simulink model "Quadcopter_Control_Simulink"  (R2022b)
settings: Solver=VariableStepAuto  StartTime=0.0  StopTime=20  RelTol=1e-3
libraries: slpidlib x6, matrix_library x4, aerolib6dof2 x1
settings Model: Creator=matho  LastModifiedBy=matho

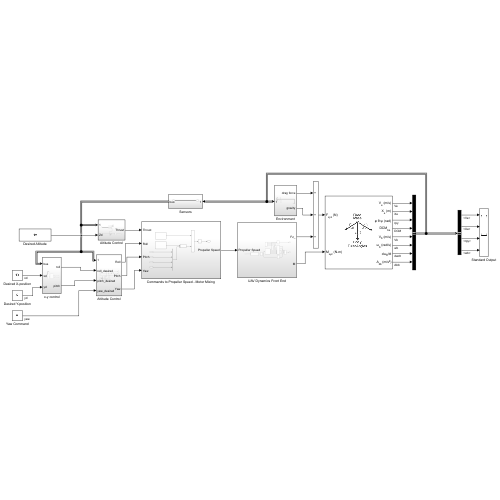
[thumbnail: Simulink's stored preview of the top-level diagram]
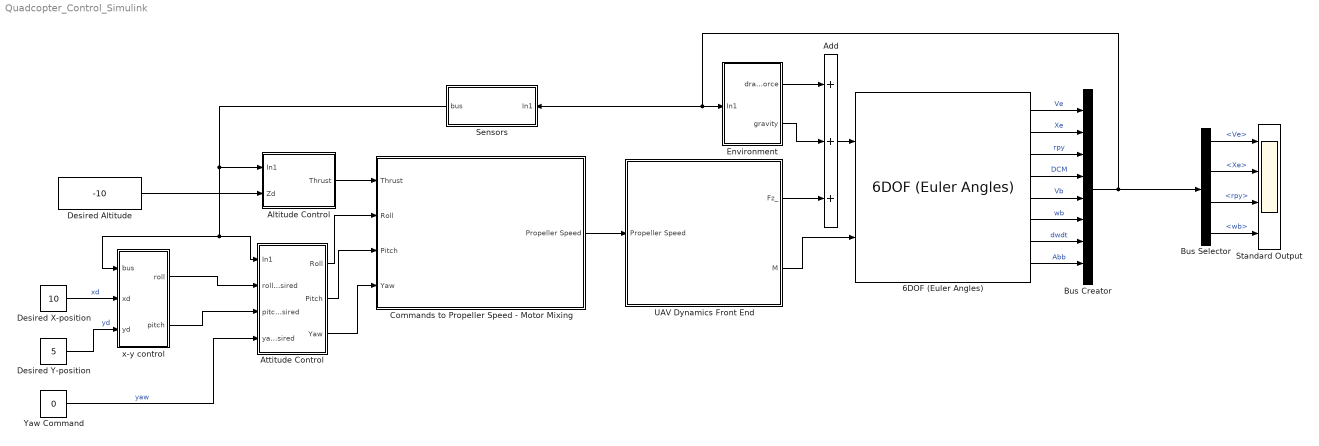
== system Quadcopter_Control_Simulink ==
  6DOF (Euler Angles) : aerolib6dof2/6DOF (Euler Angles)  units=Metric (MKS)  mtype=Fixed  rep=Euler Angles  xme_0=[0 0 0]  Vm_0=[0 0 0]  eul_0=[0 0 0]  pm_0=[0 0 0]  mass_0=1.0  mass_e=0.5  mass_f=2.0  inertia=eye(3)  inertia_e=eye(3)  inertia_f=2*eye(3)  k_quat=1.0  vre_flag=on  abi_flag=off  aMode=0  xme_statename=''  Vm_statename=''  eul_statename=''  quat_statename=''  pm_statename=''  mass_statename=''
  Add : Sum  Inputs=+++
  Altitude Control : Subsystem
  Attitude Control : Subsystem
  Bus Creator : BusCreator  Inputs=8
  Bus Selector : BusSelector  OutputSignals=Ve,Xe,rpy,wb
  "Commands to Propeller Speed - Motor Mixing " : Subsystem
  Desired Altitude : Constant  Value=-10
  Desired X-position : Constant  Value=10
  Desired Y-position : Constant  Value=5
  Environment : Subsystem
  Sensors : Subsystem
  Standard Output : Scope  NumInputPorts=4
  UAV Dynamics Front End : Subsystem
  Yaw Command : Constant  Value=0
  x-y control : Subsystem
  wires:
  6DOF (Euler Angles)/1 -> Bus Creator/1  "Ve"
  6DOF (Euler Angles)/2 -> Bus Creator/2  "Xe"
  6DOF (Euler Angles)/3 -> Bus Creator/3  "rpy"
  6DOF (Euler Angles)/4 -> Bus Creator/4  "DCM"
  6DOF (Euler Angles)/5 -> Bus Creator/5  "Vb"
  6DOF (Euler Angles)/6 -> Bus Creator/6  "wb"
  6DOF (Euler Angles)/7 -> Bus Creator/7  "dwdt"
  6DOF (Euler Angles)/8 -> Bus Creator/8  "Abb"
  Bus Selector/3 -> Standard Output/3  "<rpy>"
  Bus Selector/4 -> Standard Output/4  "<wb>"
  Bus Selector/2 -> Standard Output/2  "<Xe>"
  Bus Selector/1 -> Standard Output/1  "<Ve>"
  Add/1 -> 6DOF (Euler Angles)/1
  Bus Creator/1 -> Bus Selector/1, Sensors/1(In1), Environment/1(In1)
  Environment/1(drag force) -> Add/1
  Environment/2(gravity) -> Add/2
  UAV Dynamics Front End/2(M) -> 6DOF (Euler Angles)/2
  UAV Dynamics Front End/1(Fz_) -> Add/3
  "Commands to Propeller Speed - Motor Mixing "/1(Propeller Speed) -> UAV Dynamics Front End/1(Propeller Speed)
  Sensors/1(bus) -> Altitude Control/1(In1), Attitude Control/1(In1), x-y control/1(bus)
  Altitude Control/1(Thrust) -> "Commands to Propeller Speed - Motor Mixing "/1(Thrust)
  Attitude Control/1(Roll) -> "Commands to Propeller Speed - Motor Mixing "/2(Roll)
  Attitude Control/2(Pitch) -> "Commands to Propeller Speed - Motor Mixing "/3(Pitch)
  Attitude Control/3(Yaw) -> "Commands to Propeller Speed - Motor Mixing "/4(Yaw)
  Desired Altitude/1 -> Altitude Control/2(Zd)
  x-y control/1(roll) -> Attitude Control/2(roll_desired)
  x-y control/2(pitch) -> Attitude Control/3(pitch_desired)
  Desired X-position/1 -> x-y control/2(xd)  "xd"
  Desired Y-position/1 -> x-y control/3(yd)  "yd"
  Yaw Command/1 -> Attitude Control/4(yaw_desired)  "yaw"

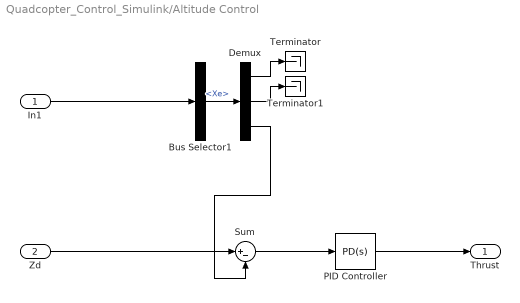
== system Quadcopter_Control_Simulink/Altitude Control ==
  In1 : Inport
  Zd : Inport  Port=2
  Bus Selector1 : BusSelector  OutputSignals=Xe
  Demux : Demux  Outputs=3
  PID Controller : slpidlib/PID Controller  Controller=PD  Form=Parallel  TimeDomain=Continuous-time  UseExternalTs=off  SampleTime=-1  IntegratorMethod=Forward Euler  FilterMethod=Forward Euler  ControllerParametersSource=internal  P=1  I=1  UseKiTs=off  D=2  N=100  UseFilter=on  TunerSelectOption=Transfer Function Based (PID Tuner App)  InitialConditionSource=internal  InitialConditionForIntegrator=0  InitialConditionForFilter=0  DifferentiatorICPrevScaledInput=0  ExternalReset=none  TrackingMode=off  Kt=1  LimitOutput=off  SatLimitsSource=internal  UpperSaturationLimit=inf  LowerSaturationLimit=-inf  LinearizeAsGain=on  AntiWindupMode=none  Kb=1  LimitIntegrator=off  UpperIntegratorSaturationLimit=inf  LowerIntegratorSaturationLimit=-inf  POutMin=[]  POutMax=[]  IOutMin=[]  IOutMax=[]  DOutMin=[]  DOutMax=[]  NOutMin=[]  NOutMax=[]  SumOutMin=[]  SumOutMax=[]  SaturationOutMin=[]  SaturationOutMax=[]  PParamMin=[]  PParamMax=[]  IParamMin=[]  IParamMax=[]  DParamMin=[]  DParamMax=[]  NParamMin=[]  NParamMax=[]  KbParamMin=[]  KbParamMax=[]  KtParamMin=[]  KtParamMax=[]  KbOutMin=[]  KbOutMax=[]  KtOutMin=[]  KtOutMax=[]  IntegratorOutMin=[]  IntegratorOutMax=[]  FilterOutMin=[]  FilterOutMax=[]  SumI1OutMin=[]  SumI1OutMax=[]  SumI2OutMin=[]  SumI2OutMax=[]  SumI3OutMin=[]  SumI3OutMax=[]  SumI4OutMin=[]  SumI4OutMax=[]  SumDOutMin=[]  SumDOutMax=[]  DifferentiatorOutMin=[]  DifferentiatorOutMax=[]  FilterDiffOutCoefMin=[]  FilterDiffOutCoefMax=[]  ReciprocalOutMin=[]  ReciprocalOutMax=[]  SumDenOutMin=[]  SumDenOutMax=[]  SumNumOutMin=[]  SumNumOutMax=[]  DivideOutMin=[]  DivideOutMax=[]  UdiffTsProdOutMin=[]  UdiffTsProdOutMax=[]  NTsProdOutMin=[]  NTsProdOutMax=[]  UintegralTsProdOutMin=[]  UintegralTsProdOutMax=[]  UngainTsProdOutMin=[]  UngainTsProdOutMax=[]  IntegratorContinuousStateAttributes=''  IntegratorStateMustResolveToSignalObject=off  IntegratorRTWStateStorageClass=Auto  FilterContinuousStateAttributes=''  FilterStateMustResolveToSignalObject=off  FilterRTWStateStorageClass=Auto  ParallelPVariant=InternalParameters  IdealPVariant=Disabled  IVariant=Disabled  DVariant=InternalParameters  IntegratorVariant=Disabled  SatVariant=Disabled  AWVariant=Disabled  PCopyVariant=Disabled  TRVariant=Disabled  FdbkBlocksVariant=Forward  IdealPFdbkVariant=Disabled  SatFdbkVariant=Disabled  DerivativeFilterVariant=ContFilter  NVariant=InternalParameters  NCopyVariant=Disabled  FilterICVariant=InternalICsFilter  IntegratorICVariant=Disabled  ExternalResetVariant=Disabled  TRSumVariant=Passthrough  SumFdbkVariant=Disabled  SumVariant=Sum_PD  TsampFilterVariant=InternalTs  TsampNgainVariant=Passthrough  TsampIntegralVariant=Disabled_SignalSpec  ExternalSaturationOutDataTypeStr=Inherit: Same as second input
  Sum : Sum  Inputs=|+-
  Terminator : Terminator
  Terminator1 : Terminator
  Thrust : Outport
  wires:
  Sum/1 -> PID Controller/1
  Demux/3 -> Sum/2
  Demux/1 -> Terminator/1
  Bus Selector1/1 -> Demux/1  "<Xe>"
  Demux/2 -> Terminator1/1
  In1/1 -> Bus Selector1/1
  PID Controller/1 -> Thrust/1
  Zd/1 -> Sum/1

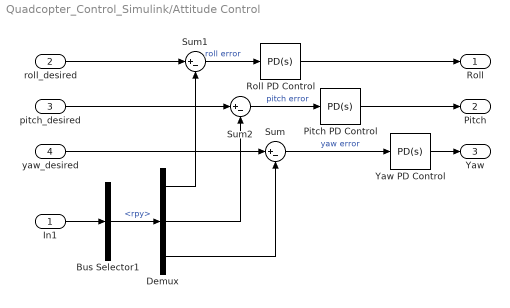
== system Quadcopter_Control_Simulink/Attitude Control ==
  In1 : Inport
  roll_desired : Inport  Port=2
  pitch_desired : Inport  Port=3
  yaw_desired : Inport  Port=4
  Bus Selector1 : BusSelector  OutputSignals=rpy
  Demux : Demux  Outputs=3
  Pitch PD Control : slpidlib/PID Controller  Controller=PD  Form=Parallel  TimeDomain=Continuous-time  UseExternalTs=off  SampleTime=-1  IntegratorMethod=Forward Euler  FilterMethod=Forward Euler  ControllerParametersSource=internal  P=1  I=1  UseKiTs=off  D=2  N=100  UseFilter=on  TunerSelectOption=Transfer Function Based (PID Tuner App)  InitialConditionSource=internal  InitialConditionForIntegrator=0  InitialConditionForFilter=0  DifferentiatorICPrevScaledInput=0  ExternalReset=none  TrackingMode=off  Kt=1  LimitOutput=off  SatLimitsSource=internal  UpperSaturationLimit=inf  LowerSaturationLimit=-inf  LinearizeAsGain=on  AntiWindupMode=none  Kb=1  LimitIntegrator=off  UpperIntegratorSaturationLimit=inf  LowerIntegratorSaturationLimit=-inf  POutMin=[]  POutMax=[]  IOutMin=[]  IOutMax=[]  DOutMin=[]  DOutMax=[]  NOutMin=[]  NOutMax=[]  SumOutMin=[]  SumOutMax=[]  SaturationOutMin=[]  SaturationOutMax=[]  PParamMin=[]  PParamMax=[]  IParamMin=[]  IParamMax=[]  DParamMin=[]  DParamMax=[]  NParamMin=[]  NParamMax=[]  KbParamMin=[]  KbParamMax=[]  KtParamMin=[]  KtParamMax=[]  KbOutMin=[]  KbOutMax=[]  KtOutMin=[]  KtOutMax=[]  IntegratorOutMin=[]  IntegratorOutMax=[]  FilterOutMin=[]  FilterOutMax=[]  SumI1OutMin=[]  SumI1OutMax=[]  SumI2OutMin=[]  SumI2OutMax=[]  SumI3OutMin=[]  SumI3OutMax=[]  SumI4OutMin=[]  SumI4OutMax=[]  SumDOutMin=[]  SumDOutMax=[]  DifferentiatorOutMin=[]  DifferentiatorOutMax=[]  FilterDiffOutCoefMin=[]  FilterDiffOutCoefMax=[]  ReciprocalOutMin=[]  ReciprocalOutMax=[]  SumDenOutMin=[]  SumDenOutMax=[]  SumNumOutMin=[]  SumNumOutMax=[]  DivideOutMin=[]  DivideOutMax=[]  UdiffTsProdOutMin=[]  UdiffTsProdOutMax=[]  NTsProdOutMin=[]  NTsProdOutMax=[]  UintegralTsProdOutMin=[]  UintegralTsProdOutMax=[]  UngainTsProdOutMin=[]  UngainTsProdOutMax=[]  IntegratorContinuousStateAttributes=''  IntegratorStateMustResolveToSignalObject=off  IntegratorRTWStateStorageClass=Auto  FilterContinuousStateAttributes=''  FilterStateMustResolveToSignalObject=off  FilterRTWStateStorageClass=Auto  ParallelPVariant=InternalParameters  IdealPVariant=Disabled  IVariant=Disabled  DVariant=InternalParameters  IntegratorVariant=Disabled  SatVariant=Disabled  AWVariant=Disabled  PCopyVariant=Disabled  TRVariant=Disabled  FdbkBlocksVariant=Forward  IdealPFdbkVariant=Disabled  SatFdbkVariant=Disabled  DerivativeFilterVariant=ContFilter  NVariant=InternalParameters  NCopyVariant=Disabled  FilterICVariant=InternalICsFilter  IntegratorICVariant=Disabled  ExternalResetVariant=Disabled  TRSumVariant=Passthrough  SumFdbkVariant=Disabled  SumVariant=Sum_PD  TsampFilterVariant=InternalTs  TsampNgainVariant=Passthrough  TsampIntegralVariant=Disabled_SignalSpec  ExternalSaturationOutDataTypeStr=Inherit: Same as second input
  Roll PD Control : slpidlib/PID Controller  Controller=PD  Form=Parallel  TimeDomain=Continuous-time  UseExternalTs=off  SampleTime=-1  IntegratorMethod=Forward Euler  FilterMethod=Forward Euler  ControllerParametersSource=internal  P=1  I=1  UseKiTs=off  D=2  N=100  UseFilter=on  TunerSelectOption=Transfer Function Based (PID Tuner App)  InitialConditionSource=internal  InitialConditionForIntegrator=0  InitialConditionForFilter=0  DifferentiatorICPrevScaledInput=0  ExternalReset=none  TrackingMode=off  Kt=1  LimitOutput=off  SatLimitsSource=internal  UpperSaturationLimit=inf  LowerSaturationLimit=-inf  LinearizeAsGain=on  AntiWindupMode=none  Kb=1  LimitIntegrator=off  UpperIntegratorSaturationLimit=inf  LowerIntegratorSaturationLimit=-inf  POutMin=[]  POutMax=[]  IOutMin=[]  IOutMax=[]  DOutMin=[]  DOutMax=[]  NOutMin=[]  NOutMax=[]  SumOutMin=[]  SumOutMax=[]  SaturationOutMin=[]  SaturationOutMax=[]  PParamMin=[]  PParamMax=[]  IParamMin=[]  IParamMax=[]  DParamMin=[]  DParamMax=[]  NParamMin=[]  NParamMax=[]  KbParamMin=[]  KbParamMax=[]  KtParamMin=[]  KtParamMax=[]  KbOutMin=[]  KbOutMax=[]  KtOutMin=[]  KtOutMax=[]  IntegratorOutMin=[]  IntegratorOutMax=[]  FilterOutMin=[]  FilterOutMax=[]  SumI1OutMin=[]  SumI1OutMax=[]  SumI2OutMin=[]  SumI2OutMax=[]  SumI3OutMin=[]  SumI3OutMax=[]  SumI4OutMin=[]  SumI4OutMax=[]  SumDOutMin=[]  SumDOutMax=[]  DifferentiatorOutMin=[]  DifferentiatorOutMax=[]  FilterDiffOutCoefMin=[]  FilterDiffOutCoefMax=[]  ReciprocalOutMin=[]  ReciprocalOutMax=[]  SumDenOutMin=[]  SumDenOutMax=[]  SumNumOutMin=[]  SumNumOutMax=[]  DivideOutMin=[]  DivideOutMax=[]  UdiffTsProdOutMin=[]  UdiffTsProdOutMax=[]  NTsProdOutMin=[]  NTsProdOutMax=[]  UintegralTsProdOutMin=[]  UintegralTsProdOutMax=[]  UngainTsProdOutMin=[]  UngainTsProdOutMax=[]  IntegratorContinuousStateAttributes=''  IntegratorStateMustResolveToSignalObject=off  IntegratorRTWStateStorageClass=Auto  FilterContinuousStateAttributes=''  FilterStateMustResolveToSignalObject=off  FilterRTWStateStorageClass=Auto  ParallelPVariant=InternalParameters  IdealPVariant=Disabled  IVariant=Disabled  DVariant=InternalParameters  IntegratorVariant=Disabled  SatVariant=Disabled  AWVariant=Disabled  PCopyVariant=Disabled  TRVariant=Disabled  FdbkBlocksVariant=Forward  IdealPFdbkVariant=Disabled  SatFdbkVariant=Disabled  DerivativeFilterVariant=ContFilter  NVariant=InternalParameters  NCopyVariant=Disabled  FilterICVariant=InternalICsFilter  IntegratorICVariant=Disabled  ExternalResetVariant=Disabled  TRSumVariant=Passthrough  SumFdbkVariant=Disabled  SumVariant=Sum_PD  TsampFilterVariant=InternalTs  TsampNgainVariant=Passthrough  TsampIntegralVariant=Disabled_SignalSpec  ExternalSaturationOutDataTypeStr=Inherit: Same as second input
  Sum : Sum  Inputs=|+-
  Sum1 : Sum  Inputs=|+-
  Sum2 : Sum  Inputs=|+-
  Yaw PD Control : slpidlib/PID Controller  Controller=PD  Form=Parallel  TimeDomain=Continuous-time  UseExternalTs=off  SampleTime=-1  IntegratorMethod=Forward Euler  FilterMethod=Forward Euler  ControllerParametersSource=internal  P=1  I=1  UseKiTs=off  D=2  N=100  UseFilter=on  TunerSelectOption=Transfer Function Based (PID Tuner App)  InitialConditionSource=internal  InitialConditionForIntegrator=0  InitialConditionForFilter=0  DifferentiatorICPrevScaledInput=0  ExternalReset=none  TrackingMode=off  Kt=1  LimitOutput=off  SatLimitsSource=internal  UpperSaturationLimit=inf  LowerSaturationLimit=-inf  LinearizeAsGain=on  AntiWindupMode=none  Kb=1  LimitIntegrator=off  UpperIntegratorSaturationLimit=inf  LowerIntegratorSaturationLimit=-inf  POutMin=[]  POutMax=[]  IOutMin=[]  IOutMax=[]  DOutMin=[]  DOutMax=[]  NOutMin=[]  NOutMax=[]  SumOutMin=[]  SumOutMax=[]  SaturationOutMin=[]  SaturationOutMax=[]  PParamMin=[]  PParamMax=[]  IParamMin=[]  IParamMax=[]  DParamMin=[]  DParamMax=[]  NParamMin=[]  NParamMax=[]  KbParamMin=[]  KbParamMax=[]  KtParamMin=[]  KtParamMax=[]  KbOutMin=[]  KbOutMax=[]  KtOutMin=[]  KtOutMax=[]  IntegratorOutMin=[]  IntegratorOutMax=[]  FilterOutMin=[]  FilterOutMax=[]  SumI1OutMin=[]  SumI1OutMax=[]  SumI2OutMin=[]  SumI2OutMax=[]  SumI3OutMin=[]  SumI3OutMax=[]  SumI4OutMin=[]  SumI4OutMax=[]  SumDOutMin=[]  SumDOutMax=[]  DifferentiatorOutMin=[]  DifferentiatorOutMax=[]  FilterDiffOutCoefMin=[]  FilterDiffOutCoefMax=[]  ReciprocalOutMin=[]  ReciprocalOutMax=[]  SumDenOutMin=[]  SumDenOutMax=[]  SumNumOutMin=[]  SumNumOutMax=[]  DivideOutMin=[]  DivideOutMax=[]  UdiffTsProdOutMin=[]  UdiffTsProdOutMax=[]  NTsProdOutMin=[]  NTsProdOutMax=[]  UintegralTsProdOutMin=[]  UintegralTsProdOutMax=[]  UngainTsProdOutMin=[]  UngainTsProdOutMax=[]  IntegratorContinuousStateAttributes=''  IntegratorStateMustResolveToSignalObject=off  IntegratorRTWStateStorageClass=Auto  FilterContinuousStateAttributes=''  FilterStateMustResolveToSignalObject=off  FilterRTWStateStorageClass=Auto  ParallelPVariant=InternalParameters  IdealPVariant=Disabled  IVariant=Disabled  DVariant=InternalParameters  IntegratorVariant=Disabled  SatVariant=Disabled  AWVariant=Disabled  PCopyVariant=Disabled  TRVariant=Disabled  FdbkBlocksVariant=Forward  IdealPFdbkVariant=Disabled  SatFdbkVariant=Disabled  DerivativeFilterVariant=ContFilter  NVariant=InternalParameters  NCopyVariant=Disabled  FilterICVariant=InternalICsFilter  IntegratorICVariant=Disabled  ExternalResetVariant=Disabled  TRSumVariant=Passthrough  SumFdbkVariant=Disabled  SumVariant=Sum_PD  TsampFilterVariant=InternalTs  TsampNgainVariant=Passthrough  TsampIntegralVariant=Disabled_SignalSpec  ExternalSaturationOutDataTypeStr=Inherit: Same as second input
  Roll : Outport
  Pitch : Outport  Port=2
  Yaw : Outport  Port=3
  wires:
  Yaw PD Control/1 -> Yaw/1
  yaw_desired/1 -> Sum/1
  Demux/3 -> Sum/2
  Demux/2 -> Sum2/2
  Demux/1 -> Sum1/2
  Bus Selector1/1 -> Demux/1  "<rpy>"
  In1/1 -> Bus Selector1/1
  Sum/1 -> Yaw PD Control/1  "yaw error"
  roll_desired/1 -> Sum1/1
  pitch_desired/1 -> Sum2/1
  Sum1/1 -> Roll PD Control/1  "roll error"
  Sum2/1 -> Pitch PD Control/1  "pitch error"
  Pitch PD Control/1 -> Pitch/1
  Roll PD Control/1 -> Roll/1

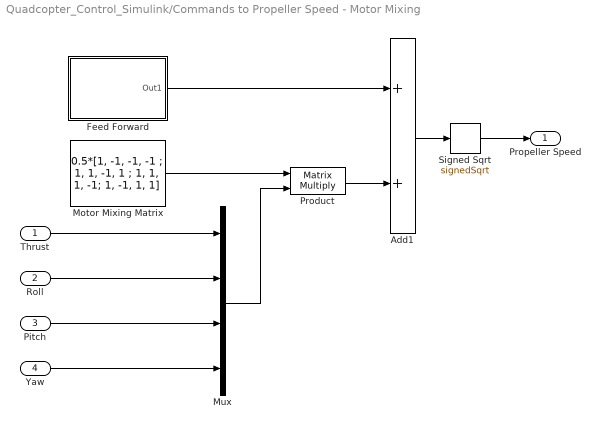
== system Quadcopter_Control_Simulink/Commands to Propeller Speed - Motor Mixing  ==
  Thrust : Inport
  Roll : Inport  Port=2
  Pitch : Inport  Port=3
  Yaw : Inport  Port=4
  Add1 : Sum
  Feed Forward : Subsystem
  Motor Mixing Matrix : Constant  Value="0.5*[1, -1, -1, -1 ; 1, 1, -1, 1 ;   1, 1, 1, -1;  1, -1, 1, 1]"  VectorParams1D=off
  Mux : Mux
  Product : Product  Multiplication=Matrix(*)
  Signed Sqrt : Sqrt  Operator=signedSqrt
  Propeller Speed : Outport
  wires:
  Feed Forward/1(Out1) -> Add1/1
  Mux/1 -> Product/2
  Pitch/1 -> Mux/3
  Product/1 -> Add1/2
  Roll/1 -> Mux/2
  Motor Mixing Matrix/1 -> Product/1
  Yaw/1 -> Mux/4
  Thrust/1 -> Mux/1
  Add1/1 -> Signed Sqrt/1
  Signed Sqrt/1 -> Propeller Speed/1

== system Quadcopter_Control_Simulink/Environment ==
  In1 : Inport
  Aerodynamic Drag : Subsystem
  Gravitational Force : Subsystem
  drag force : Outport
  gravity : Outport  Port=2
  wires:
  In1/1 -> Aerodynamic Drag/1(In1), Gravitational Force/1(In1)
  Aerodynamic Drag/1(drag force) -> drag force/1
  Gravitational Force/1(Out1) -> gravity/1

== system Quadcopter_Control_Simulink/Sensors ==
  In1 : Inport
  bus : Outport
  wires:
  In1/1 -> bus/1

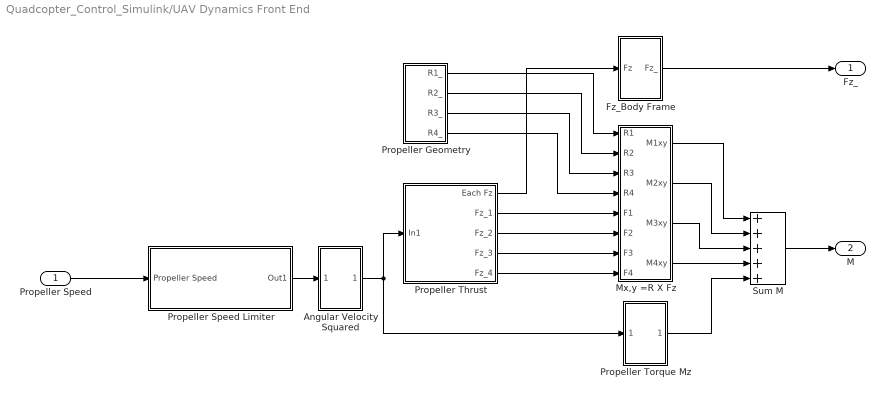
== system Quadcopter_Control_Simulink/UAV Dynamics Front End ==
  Propeller Speed : Inport
  Angular Velocity Squared : Subsystem
  Fz_Body Frame : Subsystem
  Mx,y =R X Fz : Subsystem
  Propeller Geometry : Subsystem
  Propeller Speed Limiter : Subsystem
  Propeller Thrust : Subsystem
  Propeller Torque Mz : Subsystem
  Sum M : Sum  Inputs=+++++
  Fz_ : Outport
  M : Outport  Port=2
  wires:
  Propeller Thrust/4(Fz_3) -> Mx,y =R X Fz/7(F3)
  Propeller Thrust/2(Fz_1) -> Mx,y =R X Fz/5(F1)
  Mx,y =R X Fz/4(M4xy) -> Sum M/4
  Propeller Geometry/2(R2_) -> Mx,y =R X Fz/2(R2)
  Propeller Thrust/5(Fz_4) -> Mx,y =R X Fz/8(F4)
  Mx,y =R X Fz/2(M2xy) -> Sum M/2
  Propeller Thrust/3(Fz_2) -> Mx,y =R X Fz/6(F2)
  Propeller Geometry/3(R3_) -> Mx,y =R X Fz/3(R3)
  Propeller Geometry/4(R4_) -> Mx,y =R X Fz/4(R4)
  Propeller Speed Limiter/1(Out1) -> Angular Velocity Squared/1(In1)
  Mx,y =R X Fz/3(M3xy) -> Sum M/3
  Propeller Thrust/1(Each Fz) -> Fz_Body Frame/1(Fz)
  Angular Velocity Squared/1(Out1) -> Propeller Thrust/1(In1), Propeller Torque Mz/1(In1)
  Propeller Torque Mz/1(Out1) -> Sum M/5
  Mx,y =R X Fz/1(M1xy) -> Sum M/1
  Propeller Geometry/1(R1_) -> Mx,y =R X Fz/1(R1)
  Sum M/1 -> M/1
  Propeller Speed/1 -> Propeller Speed Limiter/1(Propeller Speed)
  Fz_Body Frame/1(Fz_) -> Fz_/1

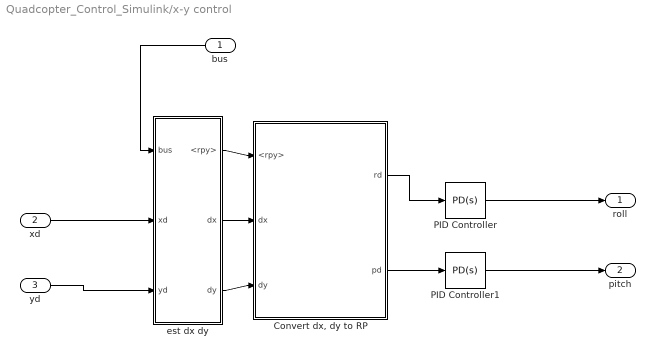
== system Quadcopter_Control_Simulink/x-y control ==
  bus : Inport
  xd : Inport  Port=2
  yd : Inport  Port=3
  "Convert dx, dy to RP" : Subsystem
  PID Controller : slpidlib/PID Controller  Controller=PD  Form=Parallel  TimeDomain=Continuous-time  UseExternalTs=off  SampleTime=-1  IntegratorMethod=Forward Euler  FilterMethod=Forward Euler  ControllerParametersSource=internal  P=1  I=1  UseKiTs=off  D=2  N=100  UseFilter=on  TunerSelectOption=Transfer Function Based (PID Tuner App)  InitialConditionSource=internal  InitialConditionForIntegrator=0  InitialConditionForFilter=0  DifferentiatorICPrevScaledInput=0  ExternalReset=none  TrackingMode=off  Kt=1  LimitOutput=on  SatLimitsSource=internal  UpperSaturationLimit=.05  LowerSaturationLimit=-.05  LinearizeAsGain=on  AntiWindupMode=none  Kb=1  LimitIntegrator=off  UpperIntegratorSaturationLimit=inf  LowerIntegratorSaturationLimit=-inf  POutMin=[]  POutMax=[]  IOutMin=[]  IOutMax=[]  DOutMin=[]  DOutMax=[]  NOutMin=[]  NOutMax=[]  SumOutMin=[]  SumOutMax=[]  SaturationOutMin=[]  SaturationOutMax=[]  PParamMin=[]  PParamMax=[]  IParamMin=[]  IParamMax=[]  DParamMin=[]  DParamMax=[]  NParamMin=[]  NParamMax=[]  KbParamMin=[]  KbParamMax=[]  KtParamMin=[]  KtParamMax=[]  KbOutMin=[]  KbOutMax=[]  KtOutMin=[]  KtOutMax=[]  IntegratorOutMin=[]  IntegratorOutMax=[]  FilterOutMin=[]  FilterOutMax=[]  SumI1OutMin=[]  SumI1OutMax=[]  SumI2OutMin=[]  SumI2OutMax=[]  SumI3OutMin=[]  SumI3OutMax=[]  SumI4OutMin=[]  SumI4OutMax=[]  SumDOutMin=[]  SumDOutMax=[]  DifferentiatorOutMin=[]  DifferentiatorOutMax=[]  FilterDiffOutCoefMin=[]  FilterDiffOutCoefMax=[]  ReciprocalOutMin=[]  ReciprocalOutMax=[]  SumDenOutMin=[]  SumDenOutMax=[]  SumNumOutMin=[]  SumNumOutMax=[]  DivideOutMin=[]  DivideOutMax=[]  UdiffTsProdOutMin=[]  UdiffTsProdOutMax=[]  NTsProdOutMin=[]  NTsProdOutMax=[]  UintegralTsProdOutMin=[]  UintegralTsProdOutMax=[]  UngainTsProdOutMin=[]  UngainTsProdOutMax=[]  IntegratorContinuousStateAttributes=''  IntegratorStateMustResolveToSignalObject=off  IntegratorRTWStateStorageClass=Auto  FilterContinuousStateAttributes=''  FilterStateMustResolveToSignalObject=off  FilterRTWStateStorageClass=Auto  ParallelPVariant=InternalParameters  IdealPVariant=Disabled  IVariant=Disabled  DVariant=InternalParameters  IntegratorVariant=Disabled  SatVariant=Enabled  AWVariant=Disabled  PCopyVariant=Disabled  TRVariant=Disabled  FdbkBlocksVariant=Forward  IdealPFdbkVariant=Disabled  SatFdbkVariant=Disabled  DerivativeFilterVariant=ContFilter  NVariant=InternalParameters  NCopyVariant=Disabled  FilterICVariant=InternalICsFilter  IntegratorICVariant=Disabled  ExternalResetVariant=Disabled  TRSumVariant=Passthrough  SumFdbkVariant=Disabled  SumVariant=Sum_PD  TsampFilterVariant=InternalTs  TsampNgainVariant=Passthrough  TsampIntegralVariant=Disabled_SignalSpec  ExternalSaturationOutDataTypeStr=Inherit: Same as second input
  PID Controller1 : slpidlib/PID Controller  Controller=PD  Form=Parallel  TimeDomain=Continuous-time  UseExternalTs=off  SampleTime=-1  IntegratorMethod=Forward Euler  FilterMethod=Forward Euler  ControllerParametersSource=internal  P=1  I=1  UseKiTs=off  D=2  N=100  UseFilter=on  TunerSelectOption=Transfer Function Based (PID Tuner App)  InitialConditionSource=internal  InitialConditionForIntegrator=0  InitialConditionForFilter=0  DifferentiatorICPrevScaledInput=0  ExternalReset=none  TrackingMode=off  Kt=1  LimitOutput=on  SatLimitsSource=internal  UpperSaturationLimit=.05  LowerSaturationLimit=-.05  LinearizeAsGain=on  AntiWindupMode=none  Kb=1  LimitIntegrator=off  UpperIntegratorSaturationLimit=inf  LowerIntegratorSaturationLimit=-inf  POutMin=[]  POutMax=[]  IOutMin=[]  IOutMax=[]  DOutMin=[]  DOutMax=[]  NOutMin=[]  NOutMax=[]  SumOutMin=[]  SumOutMax=[]  SaturationOutMin=[]  SaturationOutMax=[]  PParamMin=[]  PParamMax=[]  IParamMin=[]  IParamMax=[]  DParamMin=[]  DParamMax=[]  NParamMin=[]  NParamMax=[]  KbParamMin=[]  KbParamMax=[]  KtParamMin=[]  KtParamMax=[]  KbOutMin=[]  KbOutMax=[]  KtOutMin=[]  KtOutMax=[]  IntegratorOutMin=[]  IntegratorOutMax=[]  FilterOutMin=[]  FilterOutMax=[]  SumI1OutMin=[]  SumI1OutMax=[]  SumI2OutMin=[]  SumI2OutMax=[]  SumI3OutMin=[]  SumI3OutMax=[]  SumI4OutMin=[]  SumI4OutMax=[]  SumDOutMin=[]  SumDOutMax=[]  DifferentiatorOutMin=[]  DifferentiatorOutMax=[]  FilterDiffOutCoefMin=[]  FilterDiffOutCoefMax=[]  ReciprocalOutMin=[]  ReciprocalOutMax=[]  SumDenOutMin=[]  SumDenOutMax=[]  SumNumOutMin=[]  SumNumOutMax=[]  DivideOutMin=[]  DivideOutMax=[]  UdiffTsProdOutMin=[]  UdiffTsProdOutMax=[]  NTsProdOutMin=[]  NTsProdOutMax=[]  UintegralTsProdOutMin=[]  UintegralTsProdOutMax=[]  UngainTsProdOutMin=[]  UngainTsProdOutMax=[]  IntegratorContinuousStateAttributes=''  IntegratorStateMustResolveToSignalObject=off  IntegratorRTWStateStorageClass=Auto  FilterContinuousStateAttributes=''  FilterStateMustResolveToSignalObject=off  FilterRTWStateStorageClass=Auto  ParallelPVariant=InternalParameters  IdealPVariant=Disabled  IVariant=Disabled  DVariant=InternalParameters  IntegratorVariant=Disabled  SatVariant=Enabled  AWVariant=Disabled  PCopyVariant=Disabled  TRVariant=Disabled  FdbkBlocksVariant=Forward  IdealPFdbkVariant=Disabled  SatFdbkVariant=Disabled  DerivativeFilterVariant=ContFilter  NVariant=InternalParameters  NCopyVariant=Disabled  FilterICVariant=InternalICsFilter  IntegratorICVariant=Disabled  ExternalResetVariant=Disabled  TRSumVariant=Passthrough  SumFdbkVariant=Disabled  SumVariant=Sum_PD  TsampFilterVariant=InternalTs  TsampNgainVariant=Passthrough  TsampIntegralVariant=Disabled_SignalSpec  ExternalSaturationOutDataTypeStr=Inherit: Same as second input
  est dx dy : Subsystem
  roll : Outport
  pitch : Outport  Port=2
  wires:
  PID Controller/1 -> roll/1
  yd/1 -> est dx dy/3(yd)
  est dx dy/2(dx) -> "Convert dx, dy to RP"/2(dx)
  "Convert dx, dy to RP"/1(rd) -> PID Controller/1
  est dx dy/1(<rpy>) -> "Convert dx, dy to RP"/1(<rpy>)
  xd/1 -> est dx dy/2(xd)
  est dx dy/3(dy) -> "Convert dx, dy to RP"/3(dy)
  "Convert dx, dy to RP"/2(pd) -> PID Controller1/1
  PID Controller1/1 -> pitch/1
  bus/1 -> est dx dy/1(bus)

== system Quadcopter_Control_Simulink/Commands to Propeller Speed - Motor Mixing /Feed Forward ==
  Constant1 : Constant  Value=[1;1;1;1]
  Conversion Coefficient : Gain  Gain=9.81/4
  Direction : Gain  Gain=-1
  mass : Gain
  Out1 : Outport
  wires:
  Constant1/1 -> mass/1
  Direction/1 -> Conversion Coefficient/1
  mass/1 -> Direction/1
  Conversion Coefficient/1 -> Out1/1

== system Quadcopter_Control_Simulink/Environment/Aerodynamic Drag ==
  In1 : Inport
  Bus Selector : BusSelector  OutputSignals=Vb
  Dot Product : DotProduct  OutDataTypeStr=Inherit: Inherit via internal rule
  Product : Product
  Sqrt : Sqrt
  drag gain : Gain  Gain=-.005
  drag force : Outport
  wires:
  Dot Product/1 -> Sqrt/1
  Sqrt/1 -> Product/1
  Product/1 -> drag gain/1
  Bus Selector/1 -> Dot Product/1, Dot Product/2, Product/2  "<Vb>"
  drag gain/1 -> drag force/1
  In1/1 -> Bus Selector/1

== system Quadcopter_Control_Simulink/Environment/Gravitational Force ==
  In1 : Inport
  Gravitational Accl : Subsystem
  Mass : Gain
  Out1 : Outport
  wires:
  Mass/1 -> Out1/1
  Gravitational Accl/1(Out1) -> Mass/1
  In1/1 -> Gravitational Accl/1(In1)

== system Quadcopter_Control_Simulink/UAV Dynamics Front End/Angular Velocity Squared ==
  In1 : Inport
  Abs : Abs  SaturateOnIntegerOverflow=off
  Product : Product
  Out1 : Outport
  wires:
  In1/1 -> Product/2, Abs/1
  Abs/1 -> Product/1
  Product/1 -> Out1/1

== system Quadcopter_Control_Simulink/UAV Dynamics Front End/Fz_Body Frame ==
  Fz : Inport
  Sum of Elements : Sum  Inputs=+
  "z-vector " : Subsystem
  Fz_ : Outport
  wires:
  Sum of Elements/1 -> "z-vector "/1(Fz_in)
  "z-vector "/1(Fz_out) -> Fz_/1
  Fz/1 -> Sum of Elements/1

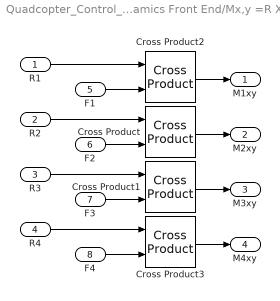
== system Quadcopter_Control_Simulink/UAV Dynamics Front End/Mx,y =R X Fz ==
  R1 : Inport
  R2 : Inport  Port=2
  R3 : Inport  Port=3
  R4 : Inport  Port=4
  F1 : Inport  Port=5
  F2 : Inport  Port=6
  F3 : Inport  Port=7
  F4 : Inport  Port=8
  Cross Product{,1..3} (4 alike) : matrix_library/Cross Product
  M1xy : Outport
  M2xy : Outport  Port=2
  M3xy : Outport  Port=3
  M4xy : Outport  Port=4
  wires:
  F4/1 -> Cross Product3/2
  Cross Product/1 -> M2xy/1
  Cross Product2/1 -> M1xy/1
  F1/1 -> Cross Product2/2
  R2/1 -> Cross Product/1
  F3/1 -> Cross Product1/2
  Cross Product3/1 -> M4xy/1
  Cross Product1/1 -> M3xy/1
  F2/1 -> Cross Product/2
  R3/1 -> Cross Product1/1
  R1/1 -> Cross Product2/1
  R4/1 -> Cross Product3/1

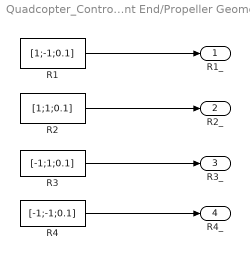
== system Quadcopter_Control_Simulink/UAV Dynamics Front End/Propeller Geometry ==
  R1 : Constant  Value=[1;-1;0.1]
  R2 : Constant  Value=[1;1;0.1]
  R3 : Constant  Value=[-1;1;0.1]
  R4 : Constant  Value=[-1;-1;0.1]
  R1_ : Outport
  R2_ : Outport  Port=2
  R3_ : Outport  Port=3
  R4_ : Outport  Port=4
  wires:
  R1/1 -> R1_/1
  R4/1 -> R4_/1
  R3/1 -> R3_/1
  R2/1 -> R2_/1

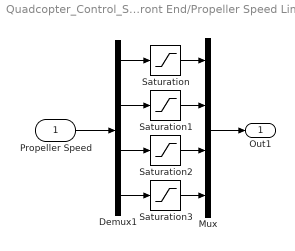
== system Quadcopter_Control_Simulink/UAV Dynamics Front End/Propeller Speed Limiter ==
  Propeller Speed : Inport
  Demux1 : Demux
  Mux : Mux
  Saturation{,1..3} (4 alike) : Saturate  UpperLimit=300  LowerLimit=-300
  Out1 : Outport
  wires:
  Demux1/2 -> Saturation1/1
  Demux1/1 -> Saturation/1
  Demux1/3 -> Saturation2/1
  Saturation2/1 -> Mux/3
  Saturation1/1 -> Mux/2
  Propeller Speed/1 -> Demux1/1
  Mux/1 -> Out1/1
  Demux1/4 -> Saturation3/1
  Saturation/1 -> Mux/1
  Saturation3/1 -> Mux/4

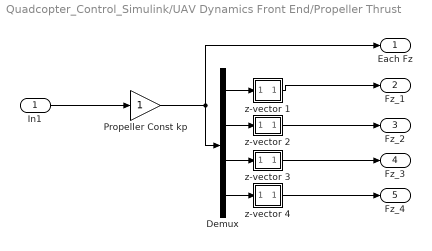
== system Quadcopter_Control_Simulink/UAV Dynamics Front End/Propeller Thrust ==
  In1 : Inport
  Demux : Demux
  Propeller Const kp : Gain
  z-vector 1 : Subsystem
  z-vector 2 : Subsystem
  z-vector 3 : Subsystem
  z-vector 4 : Subsystem
  Each Fz : Outport
  Fz_1 : Outport  Port=2
  Fz_2 : Outport  Port=3
  Fz_3 : Outport  Port=4
  Fz_4 : Outport  Port=5
  wires:
  Demux/4 -> z-vector 4/1(In1)
  Demux/1 -> z-vector 1/1(In1)
  z-vector 3/1(Out1) -> Fz_3/1
  z-vector 2/1(Out1) -> Fz_2/1
  Propeller Const kp/1 -> Each Fz/1, Demux/1
  z-vector 1/1(Out1) -> Fz_1/1
  Demux/2 -> z-vector 2/1(In1)
  Demux/3 -> z-vector 3/1(In1)
  z-vector 4/1(Out1) -> Fz_4/1
  In1/1 -> Propeller Const kp/1

== system Quadcopter_Control_Simulink/UAV Dynamics Front End/Propeller Torque Mz ==
  In1 : Inport
  Motor Torq Const km : Gain
  z-torque : Subsystem
  z-vector 5 : Subsystem
  Out1 : Outport
  wires:
  z-torque/1(Out1) -> z-vector 5/1(In1)
  Motor Torq Const km/1 -> z-torque/1(In1)
  z-vector 5/1(Out1) -> Out1/1
  In1/1 -> Motor Torq Const km/1

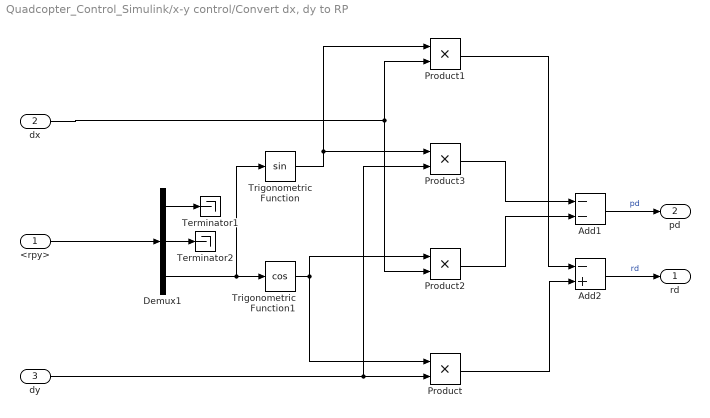
== system Quadcopter_Control_Simulink/x-y control/Convert dx, dy to RP ==
  <rpy> : Inport
  dx : Inport  Port=2
  dy : Inport  Port=3
  Add1 : Sum  Inputs=--
  Add2 : Sum  Inputs=-+
  Demux1 : Demux  Outputs=3
  Product{,1..3} (4 alike) : Product
  Terminator1 : Terminator
  Terminator2 : Terminator
  Trigonometric Function : Trigonometry
  Trigonometric Function1 : Trigonometry  Operator=cos
  rd : Outport
  pd : Outport  Port=2
  wires:
  <rpy>/1 -> Demux1/1
  Trigonometric Function1/1 -> Product/1, Product2/1
  Product1/1 -> Add2/1
  Product3/1 -> Add1/1
  Product/1 -> Add2/2
  dx/1 -> Product1/2, Product2/2
  dy/1 -> Product3/2, Product/2
  Add2/1 -> rd/1  "rd"
  Product2/1 -> Add1/2
  Demux1/1 -> Terminator1/1
  Demux1/3 -> Trigonometric Function1/1, Trigonometric Function/1
  Trigonometric Function/1 -> Product1/1, Product3/1
  Demux1/2 -> Terminator2/1
  Add1/1 -> pd/1  "pd"

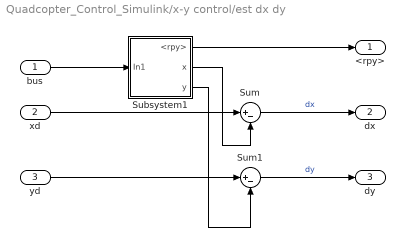
== system Quadcopter_Control_Simulink/x-y control/est dx dy ==
  bus : Inport
  xd : Inport  Port=2
  yd : Inport  Port=3
  Subsystem1 : Subsystem
  Sum : Sum  Inputs=|+-
  Sum1 : Sum  Inputs=|+-
  <rpy> : Outport
  dx : Outport  Port=2
  dy : Outport  Port=3
  wires:
  Sum/1 -> dx/1  "dx"
  Subsystem1/3(y) -> Sum1/2
  Subsystem1/2(x) -> Sum/2
  Sum1/1 -> dy/1  "dy"
  xd/1 -> Sum/1
  Subsystem1/1(<rpy>) -> <rpy>/1
  yd/1 -> Sum1/1
  bus/1 -> Subsystem1/1(In1)

== system Quadcopter_Control_Simulink/Environment/Gravitational Force/Gravitational Accl ==
  In1 : Inport
  Bus Selector : BusSelector  OutputSignals=DCM
  Constant : Constant  Value=[0;0;9.81]
  Product : Product  Multiplication=Matrix(*)
  Out1 : Outport
  wires:
  Constant/1 -> Product/2
  In1/1 -> Bus Selector/1
  Product/1 -> Out1/1
  Bus Selector/1 -> Product/1  "<DCM>"

== system Quadcopter_Control_Simulink/UAV Dynamics Front End/Fz_Body Frame/z-vector  ==
  Fz_in : Inport
  Divide : Product  Inputs=**
  az : Constant  Value=[0;0;1]
  Fz_out : Outport
  wires:
  az/1 -> Divide/1
  Divide/1 -> Fz_out/1
  Fz_in/1 -> Divide/2

== system Quadcopter_Control_Simulink/UAV Dynamics Front End/Propeller Thrust/z-vector 1 ==
  In1 : Inport
  Divide : Product  Inputs=**
  az : Constant  Value=[0;0;1]
  Out1 : Outport
  wires:
  az/1 -> Divide/1
  Divide/1 -> Out1/1
  In1/1 -> Divide/2

== system Quadcopter_Control_Simulink/UAV Dynamics Front End/Propeller Thrust/z-vector 2 ==
  In1 : Inport
  Divide : Product  Inputs=**
  az : Constant  Value=[0;0;1]
  Out1 : Outport
  wires:
  az/1 -> Divide/1
  Divide/1 -> Out1/1
  In1/1 -> Divide/2

== system Quadcopter_Control_Simulink/UAV Dynamics Front End/Propeller Thrust/z-vector 3 ==
  In1 : Inport
  Divide : Product  Inputs=**
  az : Constant  Value=[0;0;1]
  Out1 : Outport
  wires:
  az/1 -> Divide/1
  Divide/1 -> Out1/1
  In1/1 -> Divide/2

== system Quadcopter_Control_Simulink/UAV Dynamics Front End/Propeller Thrust/z-vector 4 ==
  In1 : Inport
  Divide : Product  Inputs=**
  az : Constant  Value=[0;0;1]
  Out1 : Outport
  wires:
  az/1 -> Divide/1
  Divide/1 -> Out1/1
  In1/1 -> Divide/2

== system Quadcopter_Control_Simulink/UAV Dynamics Front End/Propeller Torque Mz/z-torque ==
  In1 : Inport
  Constant : Constant  Value=[-1; 1; -1; 1]
  Product1 : Product
  Sum of Elements : Sum  Inputs=+
  Out1 : Outport
  wires:
  Constant/1 -> Product1/1
  In1/1 -> Product1/2
  Product1/1 -> Sum of Elements/1
  Sum of Elements/1 -> Out1/1

== system Quadcopter_Control_Simulink/UAV Dynamics Front End/Propeller Torque Mz/z-vector 5 ==
  In1 : Inport
  Divide : Product  Inputs=**
  az : Constant  Value=[0;0;1]
  Out1 : Outport
  wires:
  az/1 -> Divide/1
  Divide/1 -> Out1/1
  In1/1 -> Divide/2

== system Quadcopter_Control_Simulink/x-y control/est dx dy/Subsystem1 ==
  In1 : Inport
  Bus Selector : BusSelector  OutputSignals=Xe,rpy
  Demux : Demux  Outputs=3
  Terminator : Terminator
  <rpy> : Outport
  x : Outport  Port=2
  y : Outport  Port=3
  wires:
  Demux/3 -> Terminator/1
  Bus Selector/2 -> <rpy>/1  "<rpy>"
  In1/1 -> Bus Selector/1
  Demux/2 -> y/1
  Bus Selector/1 -> Demux/1  "<Xe>"
  Demux/1 -> x/1
